simulink model "ThrustControl"  (R2023a)
settings: Solver=VariableStepAuto  StartTime=0.0  StopTime=10.0  RelTol=1e-3
settings Model: Creator=aan18022  LastModifiedBy=aan18022

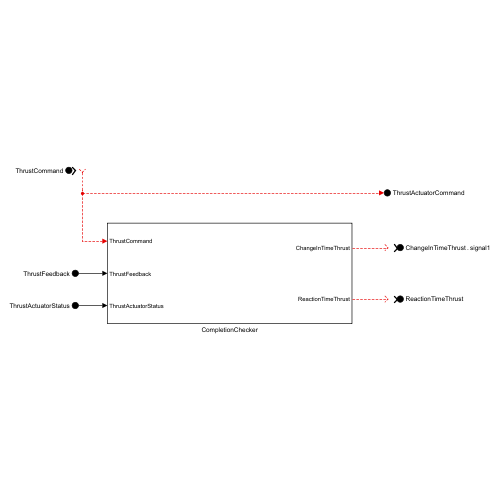
[thumbnail: Simulink's stored preview of the top-level diagram]
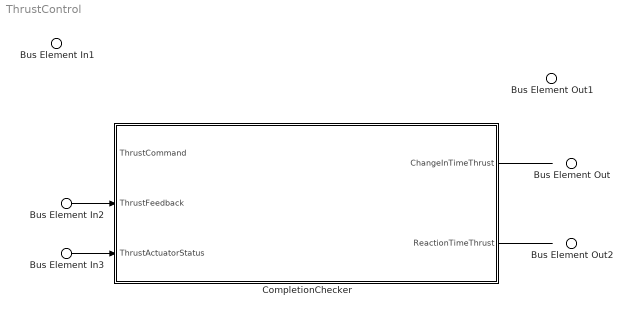
== system ThrustControl ==
  Bus Element In1 : Inport  PortName=ThrustCommand
  Bus Element In2 : Inport  Port=2  PortName=ThrustFeedback
  Bus Element In3 : Inport  Port=3  PortName=ThrustActuatorStatus
  CompletionChecker : Subsystem
  Bus Element Out1 : Outport  PortName=ThrustActuatorCommand
  Bus Element Out2 : Outport  Port=2  PortName=ReactionTimeThrust
  Bus Element Out : Outport  Port=3  PortName=ChangeInTimeThrust  Element=signal1
  wires:
  Bus Element In2/1 -> CompletionChecker/2(ThrustFeedback)
  Bus Element In3/1 -> CompletionChecker/3(ThrustActuatorStatus)
  CompletionChecker/2(ReactionTimeThrust) -> ?
  ? -> Bus Element Out1/1, CompletionChecker/1(ThrustCommand)
  CompletionChecker/1(ChangeInTimeThrust) -> ?

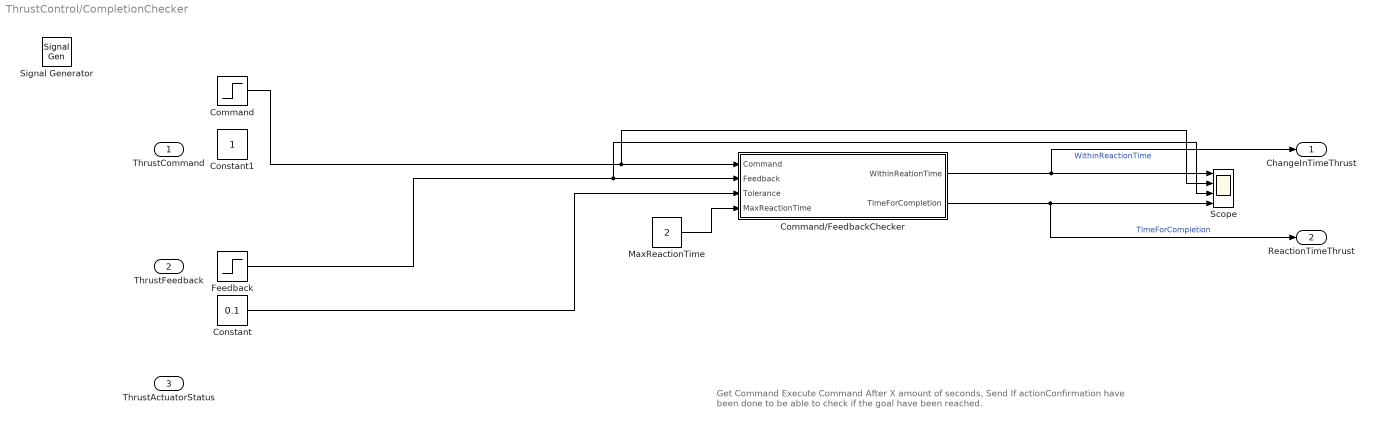
== system ThrustControl/CompletionChecker ==
  note: Get Command
      | Execute Command
      | After X amount of seconds, Send If actionConfirmation have been done to be able to check if the goal have been reached.
  ThrustCommand : Inport
  ThrustFeedback : Inport  Port=2
  ThrustActuatorStatus : Inport  Port=3
  Command : Step  Time=2  SampleTime=0
  Command/FeedbackChecker : Subsystem
  Constant : Constant  Value=0.1
  Constant1 : Constant
  Feedback : Step  Time=6  SampleTime=0
  MaxReactionTime : Constant  Value=2
  Scope : Scope  NumInputPorts=4
  Signal Generator : SignalGenerator  Frequency=0.25
  ChangeInTimeThrust : Outport
  ReactionTimeThrust : Outport  Port=2
  wires:
  Command/1 -> Scope/2, Command/FeedbackChecker/1(Command)
  Feedback/1 -> Scope/3, Command/FeedbackChecker/2(Feedback)
  Constant/1 -> Command/FeedbackChecker/3(Tolerance)
  Command/FeedbackChecker/1(WithinReationTime) -> ChangeInTimeThrust/1, Scope/1  "WithinReactionTime"
  Command/FeedbackChecker/2(TimeForCompletion) -> ReactionTimeThrust/1, Scope/4  "TimeForCompletion"
  MaxReactionTime/1 -> Command/FeedbackChecker/4(MaxReactionTime)

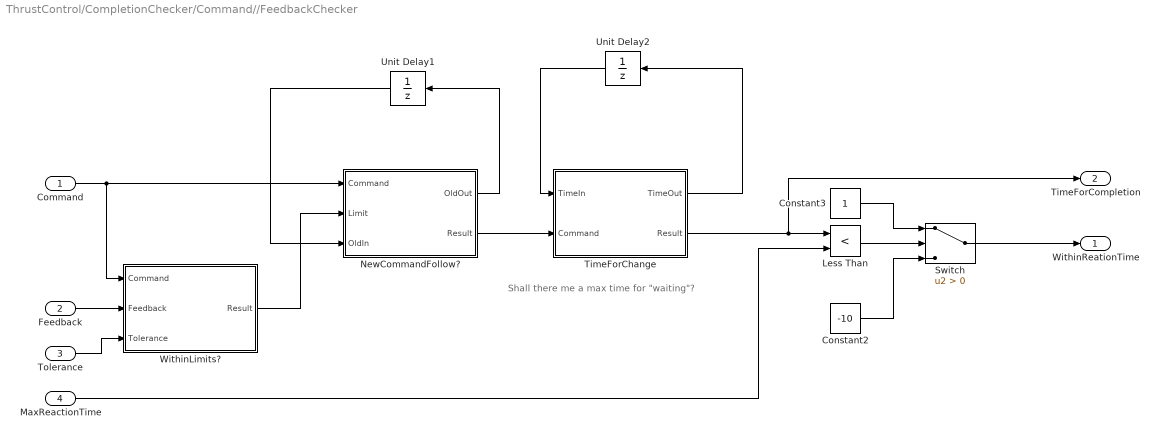
== system ThrustControl/CompletionChecker/Command//FeedbackChecker ==
  note: Shall there me a max time for "waiting"?
  Command : Inport
  Feedback : Inport  Port=2
  Tolerance : Inport  Port=3
  MaxReactionTime : Inport  Port=4
  Constant2 : Constant  Value=-10
  Constant3 : Constant
  Less Than : RelationalOperator  Operator=<  OutDataTypeStr=boolean  RndMeth=Simplest  InputSameDT=off
  NewCommandFollow? : MATLAB Function  TreatAsAtomicUnit=on
  Switch : Switch  Criteria=u2 > Threshold  SaturateOnIntegerOverflow=off  InputSameDT=off
  TimeForChange : MATLAB Function  TreatAsAtomicUnit=on
  Unit Delay1 : UnitDelay  InitialCondition=-200  SampleTime=-1  HasFrameUpgradeWarning=on
  Unit Delay2 : UnitDelay  HasFrameUpgradeWarning=on
  WithinLimits? : MATLAB Function  TreatAsAtomicUnit=on
  WithinReationTime : Outport
  TimeForCompletion : Outport  Port=2
  wires:
  TimeForChange/1(TimeOut) -> Unit Delay2/1
  Command/1 -> WithinLimits?/1(Command), NewCommandFollow?/1(Command)
  Constant2/1 -> Switch/3
  Unit Delay2/1 -> TimeForChange/1(TimeIn)
  Constant3/1 -> Switch/1
  WithinLimits?/1(Result) -> NewCommandFollow?/2(Limit)
  Less Than/1 -> Switch/2
  NewCommandFollow?/1(OldOut) -> Unit Delay1/1
  NewCommandFollow?/2(Result) -> TimeForChange/2(Command)
  Switch/1 -> WithinReationTime/1
  Feedback/1 -> WithinLimits?/2(Feedback)
  Unit Delay1/1 -> NewCommandFollow?/3(OldIn)
  Tolerance/1 -> WithinLimits?/3(Tolerance)
  TimeForChange/2(Result) -> TimeForCompletion/1, Less Than/1
  MaxReactionTime/1 -> Less Than/2

== matlab function ThrustControl/CompletionChecker/Command//FeedbackChecker/WithinLimits? ==
  data: Command input; Feedback input; Tolerance input; Result output
function Result = fcn(Command,Feedback,Tolerance)

upperLimit = Command + Tolerance;
lowerLimit = Command - Tolerance;

if (Feedback >= lowerLimit && Feedback <= upperLimit)
        Result = 1;
else
        Result = 0;
end

== matlab function ThrustControl/CompletionChecker/Command//FeedbackChecker/NewCommandFollow? ==
  data: OldOut output; Command input; Limit input; Result output; OldIn input
function [OldOut,Result]= fcn(Command,Limit,OldIn)

if OldIn == -200
    OldOut = 0;
    Result = 0;
elseif (Limit == 1)
    Result = 1;
    OldOut = Command; 
else
    Result = 0;
    OldOut = OldIn;

end

== matlab function ThrustControl/CompletionChecker/Command//FeedbackChecker/TimeForChange ==
  data: TimeIn input; TimeOut output; Command input; Result output
function [TimeOut,Result]= fcn(TimeIn, Command)

if Command == 1
    TimeOut = 0;
    Result = TimeIn;
else
    TimeOut = TimeIn+1;
    Result = 0;
end
